simulink model "lab6a_dynamics"  (R2013b)
settings: Solver=ode1  StartTime=0.0  StopTime=inf  FixedStep=0.002  RelTol=1e-3
values from neighbouring files (symbols this model uses):
  A = [0 0 0 0 1 -6.81227956989 0 15.4730759462 0 -1.49726820276 0 8.56092383613 ... (16 elements, 4x4)]    [K1_perturb.mat]    (also in K2_perturb.mat; lab6a_runner.m = [0, 1, 0, 0; osc_1_rad.mat; osc_2_rad.mat)
  B = [0 239.39947251 0 -121.533281871]    [K1_perturb.mat]    (also in K2_perturb.mat; lab6a_runner.m = [0; b_2; 0; b_4]; osc_1_rad.mat; osc_2_rad.mat)
  C = [1 0 1 0]    [K1_perturb.mat]    (also in K2_perturb.mat; lab6a_runner.m = [1, 0, 1, 0]; osc_1_rad.mat; osc_2_rad.mat)
  D = 0    [K1_perturb.mat]    (also in K2_perturb.mat; lab6a_runner.m = [0]; osc_1_rad.mat; osc_2_rad.mat)
  K = [-13.0283303674 -14.7848226904 -48.1649225129 -6.62137714178]    [K1_perturb.mat]    (also in K2_perturb.mat; lab6a_runner.m = [-13.0283303673756,-14.7848226904404,-48.1649225128586,-6.62; osc_1_rad.mat; osc_2_rad.mat)
  r = [0 0 0 0]    [K1_perturb.mat]    (also in K2_perturb.mat; lab6a_runner.m = [0; 0; 0; 0]; osc_1_rad.mat; osc_2_rad.mat)
libraries: quarc_library x2
settings Model: ExtModeTrigDuration=5000  Creator=ee128-abc  LastModifiedBy=ee128-abc
settings SolverCC: PositivePriorityOrder=on
settings RTWCC: SystemTargetFile=quarc_win64.tlc  TemplateMakefile=quarc_default_tmf  Description=QUARC Win64 Target  ProcessScript=quarc_win64_make_rtw_hook
settings STFCustomTargetCC: TargetPreCompLibLocation=C:\PROGRA~3\QUARC\lib\2013b\win64\release  GeneratePreprocessorConditionals=Disable all  CombineOutputUpdateFcns=on  GRTInterface=off  SystemTargetFile=quarc_win64.tlc
settings GRTTargetCC: TargetPreCompLibLocation=C:\PROGRA~3\QUARC\lib\2013b\win64\release  ParMdlRefBuildCompliant=off  CompOptLevelCompliant=off  ConcurrentExecutionCompliant=off  MatFileLogging=off  ExtMode=on  ExtModeMexFile=quarc_comm

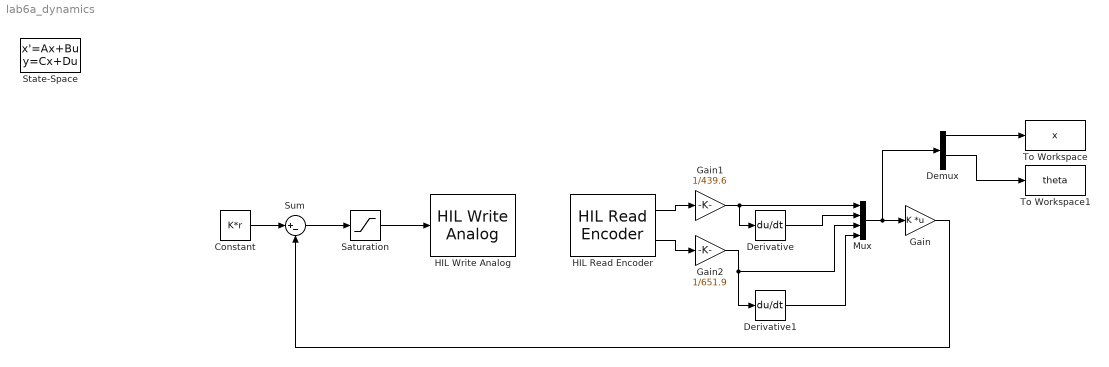
== system lab6a_dynamics ==
  Constant : Constant  Value=K*r
  Demux : Demux
  Derivative : Derivative
  Derivative1 : Derivative
  Gain : Gain  Gain=K  Multiplication=Matrix(K*u)
  Gain1 : Gain  Gain=1/439.6
  Gain2 : Gain  Gain=1/651.9
  HIL Read Encoder : quarc_library/Data Acquisition/Generic/Immediate I//O/HIL Read Encoder  object_name=unassigned  channels=[0,1]  sample_time=qc_get_step_size  active=on  vector_output=off  data_type_mode=Inherit via back propagation  data_type=double
  HIL Write Analog : quarc_library/Data Acquisition/Generic/Immediate I//O/HIL Write Analog  object_name=unassigned  channels=0  sample_time=-1  active=off  vector_input=off
  Mux : Mux
  Saturation : Saturate
  State-Space : StateSpace  A=A  B=B  C=C  D=D  X0=0
  Sum : Sum  Inputs=|+-
  To Workspace : ToWorkspace  VariableName=x  SampleTime=-1  SaveFormat=Timeseries
  To Workspace1 : ToWorkspace  VariableName=theta  SampleTime=-1  SaveFormat=Timeseries
  wires:
  Derivative1/1 -> Mux/4
  HIL Read Encoder/1 -> Gain1/1
  Gain1/1 -> Derivative/1, Mux/1
  Derivative/1 -> Mux/2
  HIL Read Encoder/2 -> Gain2/1
  Gain2/1 -> Mux/3, Derivative1/1
  Saturation/1 -> HIL Write Analog/1
  Mux/1 -> Demux/1, Gain/1
  Gain/1 -> Sum/2
  Constant/1 -> Sum/1
  Sum/1 -> Saturation/1
  Demux/1 -> To Workspace/1
  Demux/3 -> To Workspace1/1
